simulink model "sampleModel14"  (R2021b)
settings: Solver=VariableStepAuto  StartTime=0.0  StopTime=10.0  RelTol=1e-3
undefined symbols (not defined in the file or in its folder): Newton, Raphson
libraries: simulink x7, slpidlib x2
settings Model: Creator=user  LastModifiedBy=user

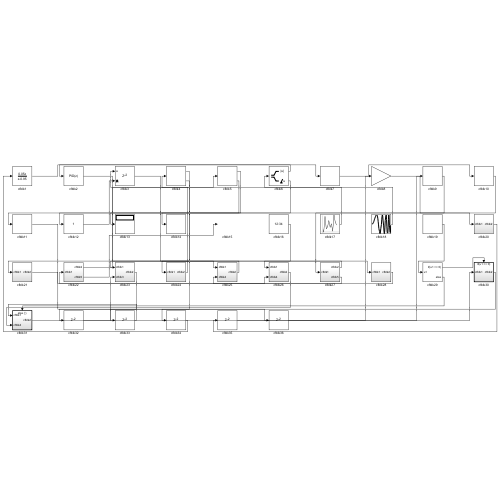
[thumbnail: Simulink's stored preview of the top-level diagram]
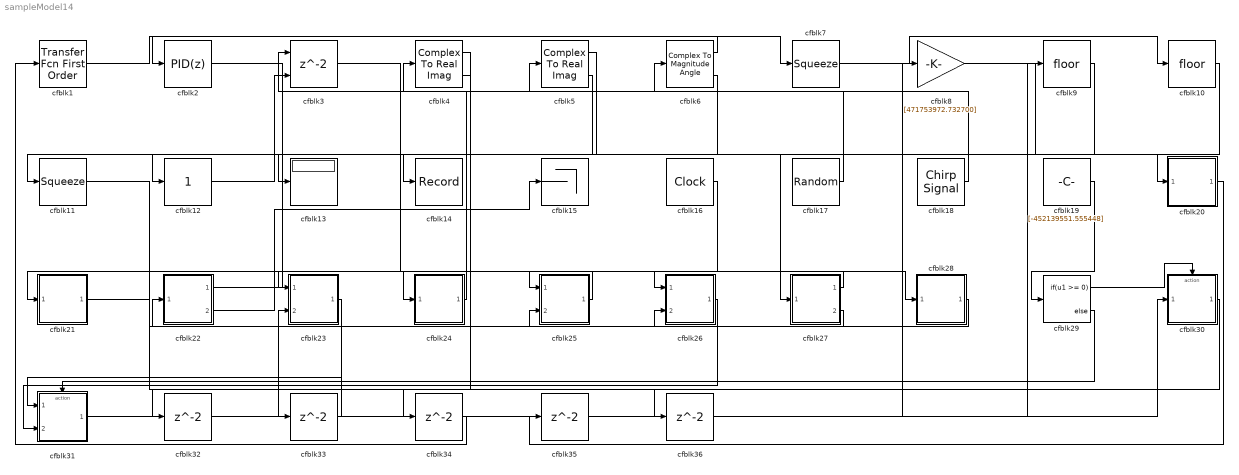
== system sampleModel14 ==
  cfblk1 : simulink/Discrete/Transfer Fcn First Order  PoleZ=0.95  ICPrevOutput=0.0  DoSatur=off
  cfblk10 : Rounding
  cfblk11 : Squeeze
  cfblk12 : simulink/Math Operations/Slider Gain  gain=1  low=0  high=2
  cfblk13 : Display
  cfblk14 : Record  FileSettingsInternal="{\"entries\":[{\"content\":{\"excelSettings\":{\"content\":{},\"type\":\"Streamout.ExcelSettings\"}},\"type\":\"Streamout.FileSettingStorage\",\"uuid\":\"8bc02c1d-e29f-4dca-9eb6-b2821a368347\"}],\"packageUris\":[\"http://schema.mathworks.com/mf0/streamout_blocks/R2020a\"],\"version\":\"1.0\"}"  SignalsInternal="{\"entries\":[{\"content\":{\"signals\":[{\"content\":{\"blockPath\":[\"sampleModel14/cfblk14\"],\"channel\":[],\"dimensions\":[1],\"domain\":\"sampleModel14/cfblk14\",\"lineColor\":\"#64d413\",\"plots\":[1],\"port\":1,\"sid\":[\"\"],\"signalID\":614,\"signalName\":\"cfblk5:2\"},\"type\":\"RecordBlkView.Signal\",\"uuid\":\"cc0fb8e1-f3dc-46df-a7d1-20c90b362ce7\"}]},\"type\":\"RecordBlkView.InputSignals\",\"uuid\":\"eb60c859-c640-48af-ab2d-2101977728c3\"}],\"packageUris\":[\"http://schema.mathworks.com/mf0/streamout_blocks/R2020a\"],\"version\":\"1.0\"}"  VisualizationBindings="{\"sparklinesplugin\":{\"info\":[{\"bindingParametersList\":[],\"subplotID\":1}]}}"
  cfblk15 : Terminator
  cfblk16 : DigitalClock
  cfblk17 : UniformRandomNumber  Minimum=[-8433829798.904942]  Maximum=[4346474114.246968]  Seed=[83224321.000000]  SampleTime=0.1
  cfblk18 : simulink/Sources/Chirp Signal  f1=[-280180877.090353]  T=[-847523904.905134]  f2=[113851091.481587]
  cfblk19 : Constant  Value=[-452139551.555448]  SampleTime=1
  cfblk2 : slpidlib/PID Controller  Controller=PID  Form=Parallel  TimeDomain=Discrete-time  UseExternalTs=off  SampleTime=1  IntegratorMethod=Forward Euler  FilterMethod=Forward Euler  ControllerParametersSource=internal  P=1  I=1  D=0  UseFilter=on  N=100  TunerSelectOption=Transfer Function Based (PID Tuner App)  InitialConditionSource=internal  InitialConditionForIntegrator=0  InitialConditionForFilter=0  DifferentiatorICPrevScaledInput=0  ExternalReset=none  TrackingMode=off  Kt=1  LimitOutput=off  SatLimitsSource=internal  UpperSaturationLimit=inf  LowerSaturationLimit=-inf  LinearizeAsGain=off  AntiWindupMode=none  Kb=1  POutMin=[]  POutMax=[]  IOutMin=[]  IOutMax=[]  DOutMin=[]  DOutMax=[]  NOutMin=[]  NOutMax=[]  SumOutMin=[]  SumOutMax=[]  SaturationOutMin=[]  SaturationOutMax=[]  PParamMin=[]  PParamMax=[]  IParamMin=[]  IParamMax=[]  DParamMin=[]  DParamMax=[]  NParamMin=[]  NParamMax=[]  KbParamMin=[]  KbParamMax=[]  KtParamMin=[]  KtParamMax=[]  KbOutMin=[]  KbOutMax=[]  KtOutMin=[]  KtOutMax=[]  IntegratorOutMin=[]  IntegratorOutMax=[]  FilterOutMin=[]  FilterOutMax=[]  SumI1OutMin=[]  SumI1OutMax=[]  SumI2OutMin=[]  SumI2OutMax=[]  SumI3OutMin=[]  SumI3OutMax=[]  SumI4OutMin=[]  SumI4OutMax=[]  SumDOutMin=[]  SumDOutMax=[]  DifferentiatorOutMin=[]  DifferentiatorOutMax=[]  FilterDiffOutCoefMin=[]  FilterDiffOutCoefMax=[]  ReciprocalOutMin=[]  ReciprocalOutMax=[]  SumDenOutMin=[]  SumDenOutMax=[]  SumNumOutMin=[]  SumNumOutMax=[]  DivideOutMin=[]  DivideOutMax=[]  UdiffTsProdOutMin=[]  UdiffTsProdOutMax=[]  NTsProdOutMin=[]  NTsProdOutMax=[]  UintegralTsProdOutMin=[]  UintegralTsProdOutMax=[]  UngainTsProdOutMin=[]  UngainTsProdOutMax=[]  IntegratorContinuousStateAttributes=''  IntegratorStateMustResolveToSignalObject=off  IntegratorRTWStateStorageClass=Auto  FilterContinuousStateAttributes=''  FilterStateMustResolveToSignalObject=off  FilterRTWStateStorageClass=Auto  ParallelPVariant=InternalParameters  IdealPVariant=Disabled  IVariant=InternalParameters  DVariant=InternalParameters  IntegratorVariant=Discrete  SatVariant=Disabled  AWVariant=Passthrough  PCopyVariant=Disabled  TRVariant=Disabled  FdbkBlocksVariant=Forward  IdealPFdbkVariant=Disabled  SatFdbkVariant=Disabled  DerivativeFilterVariant=ForwardEulerFilter  NVariant=InternalParameters  NCopyVariant=Disabled  FilterICVariant=InternalICsFilter  IntegratorICVariant=InternalICs  ExternalResetVariant=Disabled  TRSumVariant=Passthrough  SumFdbkVariant=Disabled  SumVariant=Sum_PID  TsampFilterVariant=InternalTs  TsampNgainVariant=Passthrough  TsampIntegralVariant=Passthrough  ExternalSaturationOutDataTypeStr=Inherit: Same as second input
  cfblk20 : Subsystem
  cfblk21 : Subsystem
  cfblk22 : Subsystem
  cfblk23 : Subsystem
  cfblk24 : Subsystem
  cfblk25 : Subsystem
  cfblk26 : Subsystem
  cfblk27 : Subsystem
  cfblk28 : Subsystem
  cfblk29 : If  IfExpression=u1 >= 0  SampleTime=1
  cfblk3 : Delay  ShowEnablePort=on  SampleTime=1
      settings: InputPortMap=u0,e6
  cfblk30 : Subsystem  TreatAsAtomicUnit=on
  cfblk31 : Subsystem  TreatAsAtomicUnit=on
  cfblk{32..36} (5 alike) : Delay  SampleTime=1
  cfblk4 : ComplexToRealImag
  cfblk5 : ComplexToRealImag
  cfblk6 : ComplexToMagnitudeAngle
  cfblk7 : Squeeze
  cfblk8 : Gain  Gain=[471753972.732700]
  cfblk9 : Rounding
  wires:
  cfblk8/1 -> cfblk20/1(cfblk1)
  cfblk22/1(cfblk2) -> cfblk5/1
  cfblk25/1(cfblk2) -> cfblk24/1(cfblk1)
  cfblk7/1 -> cfblk10/1
  cfblk27/1(cfblk2) -> cfblk26/1(cfblk1)
  cfblk19/1 -> cfblk29/1
  cfblk6/1 -> cfblk2/1
  cfblk10/1 -> cfblk27/1(cfblk1)
  cfblk27/2(cfblk5) -> cfblk22/1(cfblk1)
  cfblk18/1 -> cfblk6/1
  cfblk1/1 -> cfblk7/1
  cfblk2/1 -> cfblk25/1(cfblk1)
  cfblk6/2 -> cfblk13/1
  cfblk24/1(cfblk2) -> cfblk4/1
  cfblk3/1 -> cfblk28/1(cfblk1)
  cfblk28/1(cfblk2) -> cfblk25/2(cfblk4)
  cfblk17/1 -> cfblk3/1
  cfblk21/1(cfblk2) -> cfblk26/2(cfblk4)
  cfblk26/1(cfblk2) -> cfblk31/2(cfblk4)
  cfblk4/1 -> cfblk23/1(cfblk1)
  cfblk5/1 -> cfblk12/1
  cfblk16/1 -> cfblk21/1(cfblk1)
  cfblk31/1(cfblk2) -> cfblk23/2(cfblk3)
  cfblk9/1 -> cfblk11/1
  cfblk12/1 -> cfblk3/2
  cfblk5/2 -> cfblk14/1
  cfblk22/2(cfblk5) -> cfblk15/1
  cfblk29/1 -> cfblk30/Action
  cfblk29/2 -> cfblk31/Action
  cfblk23/1(cfblk2) -> cfblk32/1
  cfblk32/1 -> cfblk30/1(cfblk1)
  cfblk30/1(cfblk2) -> cfblk33/1
  cfblk33/1 -> cfblk31/1(cfblk1)
  cfblk4/2 -> cfblk34/1
  cfblk34/1 -> cfblk1/1
  cfblk20/1(cfblk2) -> cfblk35/1
  cfblk35/1 -> cfblk8/1
  cfblk11/1 -> cfblk36/1
  cfblk36/1 -> cfblk9/1

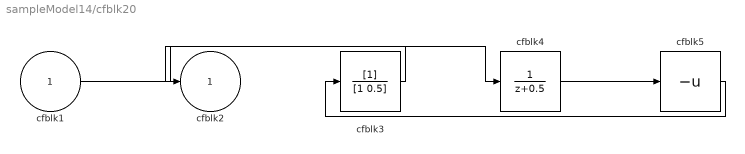
== system sampleModel14/cfblk20 ==
  cfblk1 : Inport
  cfblk3 : DiscreteFilter  SampleTime=1
  cfblk4 : DiscreteTransferFcn  SampleTime=1
  cfblk5 : UnaryMinus
  cfblk2 : Outport
  wires:
  cfblk1/1 -> cfblk4/1
  cfblk5/1 -> cfblk3/1
  cfblk4/1 -> cfblk5/1
  cfblk3/1 -> cfblk2/1

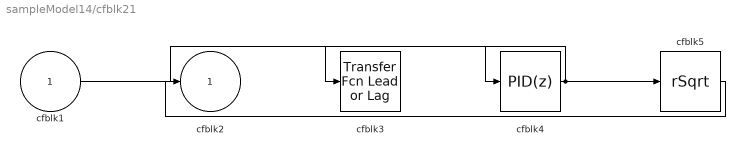
== system sampleModel14/cfblk21 ==
  cfblk1 : Inport
  cfblk3 : simulink/Discrete/Transfer Fcn Lead or Lag  PoleZ=0.95  ZeroZ=0.75  ICPrevOutput=0.0  ICPrevInput=0.0  DoSatur=off
      settings: SourceProductBaseCode=SL
  cfblk4 : slpidlib/PID Controller  Controller=PID  Form=Parallel  TimeDomain=Discrete-time  UseExternalTs=off  SampleTime=1  IntegratorMethod=Forward Euler  FilterMethod=Forward Euler  ControllerParametersSource=internal  P=1  I=1  D=0  UseFilter=on  N=100  TunerSelectOption=Transfer Function Based (PID Tuner App)  InitialConditionSource=internal  InitialConditionForIntegrator=0  InitialConditionForFilter=0  DifferentiatorICPrevScaledInput=0  ExternalReset=none  TrackingMode=off  Kt=1  LimitOutput=off  SatLimitsSource=internal  UpperSaturationLimit=inf  LowerSaturationLimit=-inf  LinearizeAsGain=off  AntiWindupMode=none  Kb=1  POutMin=[]  POutMax=[]  IOutMin=[]  IOutMax=[]  DOutMin=[]  DOutMax=[]  NOutMin=[]  NOutMax=[]  SumOutMin=[]  SumOutMax=[]  SaturationOutMin=[]  SaturationOutMax=[]  PParamMin=[]  PParamMax=[]  IParamMin=[]  IParamMax=[]  DParamMin=[]  DParamMax=[]  NParamMin=[]  NParamMax=[]  KbParamMin=[]  KbParamMax=[]  KtParamMin=[]  KtParamMax=[]  KbOutMin=[]  KbOutMax=[]  KtOutMin=[]  KtOutMax=[]  IntegratorOutMin=[]  IntegratorOutMax=[]  FilterOutMin=[]  FilterOutMax=[]  SumI1OutMin=[]  SumI1OutMax=[]  SumI2OutMin=[]  SumI2OutMax=[]  SumI3OutMin=[]  SumI3OutMax=[]  SumI4OutMin=[]  SumI4OutMax=[]  SumDOutMin=[]  SumDOutMax=[]  DifferentiatorOutMin=[]  DifferentiatorOutMax=[]  FilterDiffOutCoefMin=[]  FilterDiffOutCoefMax=[]  ReciprocalOutMin=[]  ReciprocalOutMax=[]  SumDenOutMin=[]  SumDenOutMax=[]  SumNumOutMin=[]  SumNumOutMax=[]  DivideOutMin=[]  DivideOutMax=[]  UdiffTsProdOutMin=[]  UdiffTsProdOutMax=[]  NTsProdOutMin=[]  NTsProdOutMax=[]  UintegralTsProdOutMin=[]  UintegralTsProdOutMax=[]  UngainTsProdOutMin=[]  UngainTsProdOutMax=[]  IntegratorContinuousStateAttributes=''  IntegratorStateMustResolveToSignalObject=off  IntegratorRTWStateStorageClass=Auto  FilterContinuousStateAttributes=''  FilterStateMustResolveToSignalObject=off  FilterRTWStateStorageClass=Auto  ParallelPVariant=InternalParameters  IdealPVariant=Disabled  IVariant=InternalParameters  DVariant=InternalParameters  IntegratorVariant=Discrete  SatVariant=Disabled  AWVariant=Passthrough  PCopyVariant=Disabled  TRVariant=Disabled  FdbkBlocksVariant=Forward  IdealPFdbkVariant=Disabled  SatFdbkVariant=Disabled  DerivativeFilterVariant=ForwardEulerFilter  NVariant=InternalParameters  NCopyVariant=Disabled  FilterICVariant=InternalICsFilter  IntegratorICVariant=InternalICs  ExternalResetVariant=Disabled  TRSumVariant=Passthrough  SumFdbkVariant=Disabled  SumVariant=Sum_PID  TsampFilterVariant=InternalTs  TsampNgainVariant=Passthrough  TsampIntegralVariant=Passthrough  ExternalSaturationOutDataTypeStr=Inherit: Same as second input
  cfblk5 : Sqrt  Operator=rSqrt  AlgorithmType=Newton-Raphson  SaturateOnIntegerOverflow=on
  cfblk2 : Outport
  wires:
  cfblk4/1 -> cfblk5/1, cfblk3/1
  cfblk1/1 -> cfblk4/1
  cfblk5/1 -> cfblk2/1

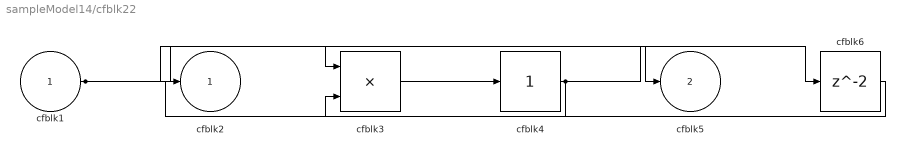
== system sampleModel14/cfblk22 ==
  cfblk1 : Inport
  cfblk3 : Product
  cfblk4 : simulink/Math Operations/Slider Gain  gain=1  low=0  high=2
  cfblk6 : Delay  SampleTime=1
  cfblk2 : Outport
  cfblk5 : Outport  Port=2
  wires:
  cfblk1/1 -> cfblk3/1, cfblk5/1
  cfblk4/1 -> cfblk2/1, cfblk6/1
  cfblk3/1 -> cfblk4/1
  cfblk6/1 -> cfblk3/2

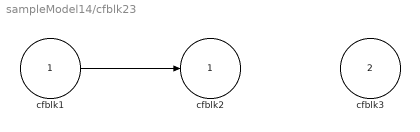
== system sampleModel14/cfblk23 ==
  cfblk1 : Inport
  cfblk3 : Inport  Port=2
  cfblk2 : Outport
  wires:
  cfblk1/1 -> cfblk2/1

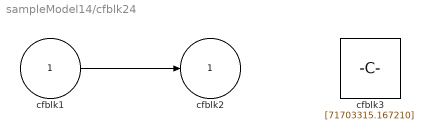
== system sampleModel14/cfblk24 ==
  cfblk1 : Inport
  cfblk3 : Constant  Value=[71703315.167210]  SampleTime=1
  cfblk2 : Outport
  wires:
  cfblk1/1 -> cfblk2/1

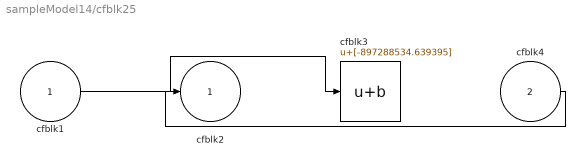
== system sampleModel14/cfblk25 ==
  cfblk1 : Inport
  cfblk4 : Inport  Port=2
  cfblk3 : Bias  Bias=[-897288534.639395]
  cfblk2 : Outport
  wires:
  cfblk1/1 -> cfblk3/1
  cfblk4/1 -> cfblk2/1

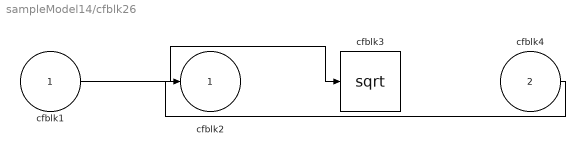
== system sampleModel14/cfblk26 ==
  cfblk1 : Inport
  cfblk4 : Inport  Port=2
  cfblk3 : Sqrt  SaturateOnIntegerOverflow=on
  cfblk2 : Outport
  wires:
  cfblk1/1 -> cfblk3/1
  cfblk4/1 -> cfblk2/1

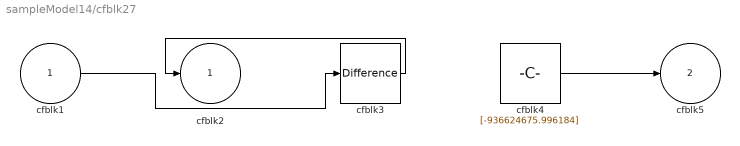
== system sampleModel14/cfblk27 ==
  cfblk1 : Inport
  cfblk3 : simulink/Discrete/Difference  ICPrevInput=0.0  OutMin=[]  OutMax=[]  OutDataTypeStr=Inherit: Inherit via back propagation  OutDataType=fixdt(1, 16)  OutScaling=2^-10  DoSatur=off
  cfblk4 : Constant  Value=[-936624675.996184]  SampleTime=1
  cfblk2 : Outport
  cfblk5 : Outport  Port=2
  wires:
  cfblk3/1 -> cfblk2/1
  cfblk4/1 -> cfblk5/1
  cfblk1/1 -> cfblk3/1

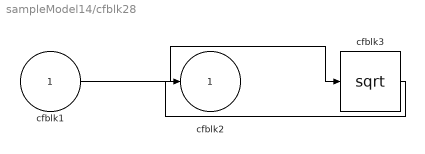
== system sampleModel14/cfblk28 ==
  cfblk1 : Inport
  cfblk3 : Sqrt  SaturateOnIntegerOverflow=on
  cfblk2 : Outport
  wires:
  cfblk1/1 -> cfblk3/1
  cfblk3/1 -> cfblk2/1

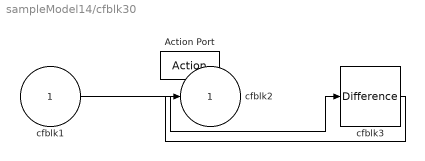
== system sampleModel14/cfblk30 ==
  cfblk1 : Inport
  Action Port : ActionPort  ActionPortLabel=if(u1 >= 0)
  cfblk3 : simulink/Discrete/Difference  ICPrevInput=0.0  OutMin=[]  OutMax=[]  OutDataTypeStr=Inherit: Inherit via back propagation  OutDataType=fixdt(1, 16)  OutScaling=2^-10  DoSatur=off
  cfblk2 : Outport
  wires:
  cfblk1/1 -> cfblk3/1
  cfblk3/1 -> cfblk2/1

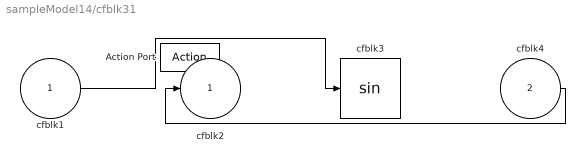
== system sampleModel14/cfblk31 ==
  cfblk1 : Inport
  cfblk4 : Inport  Port=2
  Action Port : ActionPort  ActionPortLabel=else
  cfblk3 : Trigonometry
  cfblk2 : Outport
  wires:
  cfblk4/1 -> cfblk2/1
  cfblk1/1 -> cfblk3/1
